simulink model "ArduinoTests"  (R2015b)
settings: Solver=FixedStepAuto  StartTime=0.0  StopTime=100.0  RelTol=1e-3
libraries: arduinolib x13
settings Model: SimulationMode=external  ExtModeTrigDuration=2  Creator=Joern  LastModifiedBy=Joern
settings OptimizationCC: OptimizeModelRefInitCode=on  LifeSpan=1  MaxStackSize=64
settings HardwareCC: ProdBitPerInt=16  ProdBitPerPointer=16  ProdLargestAtomicFloat=None  ProdWordSize=8  ProdHWDeviceType=Atmel->AVR
settings RTWCC: SystemTargetFile=ert.tlc  TemplateMakefile=ert_default_tmf  Description=Embedded Coder  Toolchain=Arduino AVR v1.6.1  BuildConfiguration=Faster Runs
settings CodeAppCC: IgnoreCustomStorageClasses=off
settings ERTTargetCC: GenerateSampleERTMain=on  SupportContinuousTime=on  SupportVariableSizeSignals=on

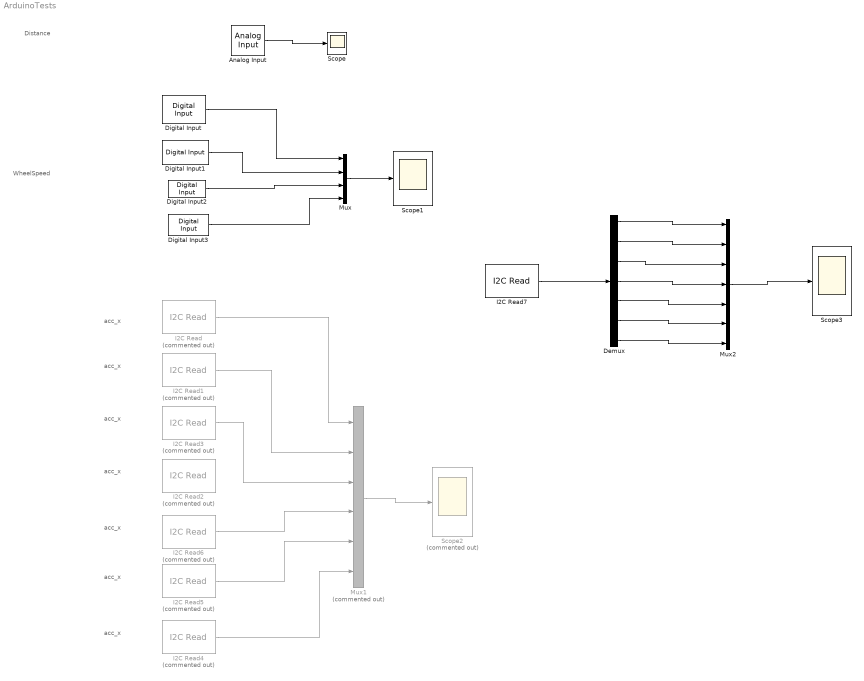
== system ArduinoTests ==
  note: acc_x
  note: WheelSpeed
  note: Distance
  note: acc_x
  note: acc_x
  note: acc_x
  note: acc_x
  note: acc_x
  note: acc_x
  Analog Input : arduinolib/Analog Input  pinNumber=6  sampleTime=0.1  blockPlatform=arduino
  Demux : Demux  Outputs=7
  Digital Input : arduinolib/Digital Input  pinNumber=18  sampleTime=0.01  blockPlatform=arduino
  Digital Input1 : arduinolib/Digital Input  pinNumber=19  sampleTime=0.01  blockPlatform=arduino
  Digital Input2 : arduinolib/Digital Input  pinNumber=2  sampleTime=0.01  blockPlatform=arduino
  Digital Input3 : arduinolib/Digital Input  pinNumber=3  sampleTime=0.01  blockPlatform=arduino
  I2C Read : arduinolib/I2C Read  Commented=on  SlaveAddress_=hex2dec( '68' )  RegisterAddressEnable=on  RegisterAddress_=hex2dec( '3B' )  Datatype=uint16  ByteOrder=Little Endian  Datalength_=1  SampleTime_=1  blockPlatform=arduino
  I2C Read1 : arduinolib/I2C Read  Commented=on  SlaveAddress_=hex2dec( '68' )  RegisterAddressEnable=on  RegisterAddress_=hex2dec( '3D' )  Datatype=uint16  ByteOrder=Little Endian  Datalength_=1  SampleTime_=1  blockPlatform=arduino
  I2C Read2 : arduinolib/I2C Read  Commented=on  SlaveAddress_=hex2dec( '68' )  RegisterAddressEnable=on  RegisterAddress_=hex2dec( '41' )  Datatype=uint16  ByteOrder=Little Endian  Datalength_=1  SampleTime_=1  blockPlatform=arduino
  I2C Read3 : arduinolib/I2C Read  Commented=on  SlaveAddress_=hex2dec( '68' )  RegisterAddressEnable=on  RegisterAddress_=hex2dec( '3F' )  Datatype=uint16  ByteOrder=Little Endian  Datalength_=1  SampleTime_=1  blockPlatform=arduino
  I2C Read4 : arduinolib/I2C Read  Commented=on  SlaveAddress_=hex2dec( '68' )  RegisterAddressEnable=on  RegisterAddress_=hex2dec( '47' )  Datatype=uint16  ByteOrder=Little Endian  Datalength_=1  SampleTime_=1  blockPlatform=arduino
  I2C Read5 : arduinolib/I2C Read  Commented=on  SlaveAddress_=hex2dec( '68' )  RegisterAddressEnable=on  RegisterAddress_=hex2dec( '45' )  Datatype=uint16  ByteOrder=Little Endian  Datalength_=1  SampleTime_=1  blockPlatform=arduino
  I2C Read6 : arduinolib/I2C Read  Commented=on  SlaveAddress_=hex2dec( '68' )  RegisterAddressEnable=on  RegisterAddress_=hex2dec( '43' )  Datatype=uint16  ByteOrder=Little Endian  Datalength_=1  SampleTime_=1  blockPlatform=arduino
  I2C Read7 : arduinolib/I2C Read  SlaveAddress_=hex2dec( '68' )  RegisterAddressEnable=on  RegisterAddress_=hex2dec( '3B' )  Datatype=uint16  ByteOrder=Little Endian  Datalength_=14  SampleTime_=0.01  blockPlatform=arduino
  Mux : Mux
  Mux1 : Mux  Commented=on  Inputs=6
  Mux2 : Mux  Inputs=7
  Scope : Scope
  Scope1 : Scope
  Scope2 : Scope  Commented=on
  Scope3 : Scope
  wires:
  Analog Input/1 -> Scope/1
  Mux/1 -> Scope1/1
  Digital Input/1 -> Mux/1
  Digital Input1/1 -> Mux/2
  Digital Input2/1 -> Mux/3
  Digital Input3/1 -> Mux/4
  Mux1/1 -> Scope2/1
  I2C Read/1 -> Mux1/1
  I2C Read1/1 -> Mux1/2
  I2C Read3/1 -> Mux1/3
  I2C Read6/1 -> Mux1/4
  I2C Read5/1 -> Mux1/5
  I2C Read4/1 -> Mux1/6
  I2C Read7/1 -> Demux/1
  Demux/1 -> Mux2/1
  Demux/2 -> Mux2/2
  Demux/3 -> Mux2/3
  Demux/4 -> Mux2/4
  Demux/5 -> Mux2/5
  Demux/6 -> Mux2/6
  Demux/7 -> Mux2/7
  Mux2/1 -> Scope3/1
